simulink model "ThreePhaseDiodeRectifier"  (R2018a)
settings: Solver=VariableStepAuto  StartTime=0.0  StopTime=0.05  MaxStep=1e-5  RelTol=1e-3
libraries: powerlib x15, powerlib_meascontrol x1
settings Model: Creator=oguna  LastModifiedBy=Emre Deniz
settings DebuggingCC: LibraryContextMissingDiagnostic=warning
settings SFSimCC: SimUseLocalCustomCode=on
settings RTWCC: RTWUseLocalCustomCode=on

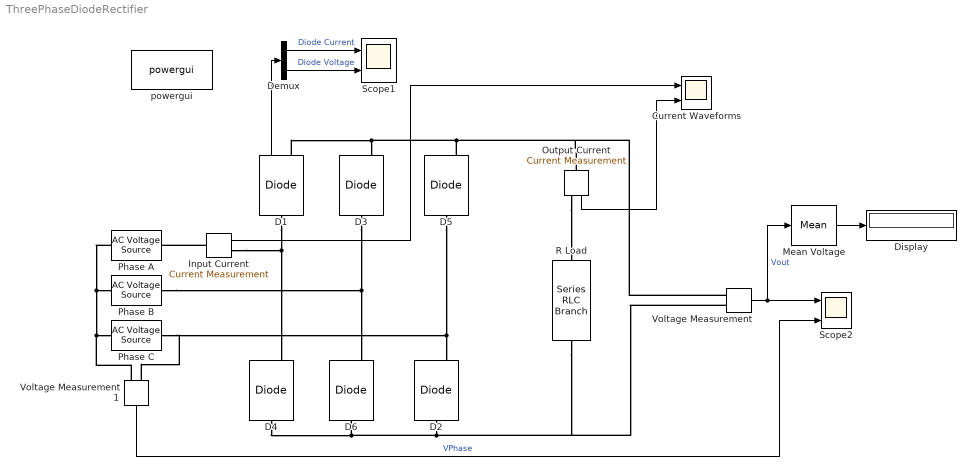
== system ThreePhaseDiodeRectifier ==
  Current Waveforms : Scope  NumInputPorts=2
  D{1..6} (6 alike) : powerlib/Power Electronics/Diode  Ron=0  Lon=0  Vf=0  IC=0  UseSnubber=0  Rs=inf  Cs=0  Measurements=on
  Demux : Demux  Outputs=2
  Display : Display
  Input Current : powerlib/Measurements/Current Measurement  PhasorSimulation=off  OutputType=Complex  PSBequivalent=0
  Mean Voltage : powerlib_meascontrol/Measurements/Mean  Freq=50  Vinit=0  Ts=0
  Output Current : powerlib/Measurements/Current Measurement  PhasorSimulation=off  OutputType=Complex  PSBequivalent=0
  Phase A : powerlib/Electrical Sources/AC Voltage Source  Amplitude=100*sqrt(2)  Phase=0  Frequency=50  SampleTime=0  Measurements=None  BusType=swing  Pref=10e3  Qref=0  Qmin=-inf  Qmax=+inf
  Phase B : powerlib/Electrical Sources/AC Voltage Source  Amplitude=100*sqrt(2)  Phase=-120  Frequency=50  SampleTime=0  Measurements=None  BusType=swing  Pref=10e3  Qref=0  Qmin=-inf  Qmax=+inf
  Phase C : powerlib/Electrical Sources/AC Voltage Source  Amplitude=100*sqrt(2)  Phase=120  Frequency=50  SampleTime=0  Measurements=None  BusType=swing  Pref=10e3  Qref=0  Qmin=-inf  Qmax=+inf
  R Load : powerlib/Elements/Series RLC Branch  LConnTagsString=__new0  RConnTagsString=__new0  BranchType=R  Resistance=1  Inductance=1e-3  SetiL0=off  InitialCurrent=0  Capacitance=1e-6  Setx0=off  InitialVoltage=0  Measurements=None
  Scope1 : Scope  NumInputPorts=2
  Scope2 : Scope  NumInputPorts=2
  Voltage Measurement : powerlib/Measurements/Voltage Measurement  PhasorSimulation=off  OutputType=Complex  PSBequivalent=0
  Voltage Measurement1 : powerlib/Measurements/Voltage Measurement  PhasorSimulation=off  OutputType=Complex  PSBequivalent=0
  powergui : powerlib/powergui  Priority=1  SimulationMode=Continuous  SampleTime=50e-6  frequency=60  Iterations=50  frequencyindice=50  Pbase=100e6  ErrMax=1e-4  UnitsV=kV  UnitsW=MW  buscounter=0  FunctionMessages=off  echomessages=off  EnableUseOfTLC=off  CurrentSourceSwitches=off  DisableSnubberDevices=off  DisableRonSwitches=off  DisableVfSwitches=off  DisplayEquations=off  SolverType=Tustin/Backward Euler (TBE)  Interpol=off  ExternalGateDelay=off  methode=off  Ts=100  x0status=blocks  SPID=on  SwTol=0  HookPort=off  RestoreLinks=warning  ResistiveCurrentMeasurement=off  Frange=[0:2:500]  Ylog=off  Xlog=on  ShowGrid=off  save=off  variable=ZData  structure=0  ZoomFFT=off  StartTime=0.0  cycles=1  DisplayStyle=1  fundamental=60  FreqAxis=off  MaxFrequency=1000  frequencyindicesteady=1  RmsSteady=1  display=off
  wires:
  Voltage Measurement/1 -> Scope2/1, Mean Voltage/1  "Vout"
  Mean Voltage/1 -> Display/1
  D1/1 -> Demux/1
  Demux/2 -> Scope1/2  "Diode Voltage"
  Demux/1 -> Scope1/1  "Diode Current"
  Voltage Measurement1/1 -> Scope2/2  "VPhase"
  Input Current/1 -> Current Waveforms/1
  Output Current/1 -> Current Waveforms/2
  connections:
  Phase A/LConn1 -- Voltage Measurement1/LConn2 -- Phase C/LConn1 -- Phase B/LConn1
  D1/LConn1 -- Input Current/RConn1 -- D4/RConn1
  D3/LConn1 -- Phase B/RConn1 -- D6/RConn1
  D5/LConn1 -- Voltage Measurement1/LConn1 -- Phase C/RConn1 -- D2/RConn1
  D1/RConn1 -- Output Current/LConn1 -- Voltage Measurement/LConn1 -- D5/RConn1 -- D3/RConn1
  D4/LConn1 -- Voltage Measurement/LConn2 -- R Load/RConn1 -- D2/LConn1 -- D6/LConn1
  Output Current/RConn1 -- R Load/LConn1
  Input Current/LConn1 -- Phase A/RConn1
